simulink model "OpenLoopBallandBeam"  (R2019a)
settings: Solver=VariableStepAuto  StartTime=0.0  StopTime=10.0  RelTol=1e-3
values from neighbouring files (symbols this model uses):
  A = [0   1   0   0 ... (first row only)    [BallandBeamModeling.m]
  B = [0;  b1; 0;  0]    [BallandBeamModeling.m]
undefined symbols (not defined in the file or in its folder): K_servo
settings Model: Creator=xde12  LastModifiedBy=xde12

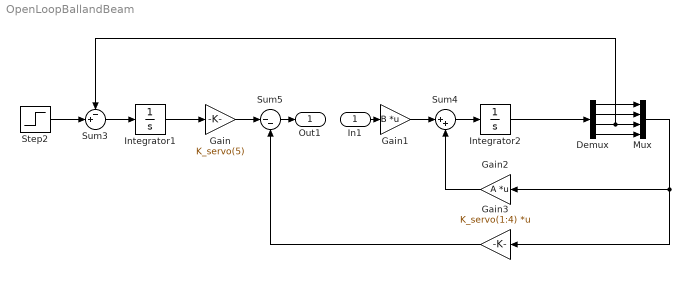
== system OpenLoopBallandBeam ==
  In1 : Inport
  Demux : Demux
  Gain : Gain  Gain=K_servo(5)
  Gain1 : Gain  Gain=B  Multiplication=Matrix(K*u)
  Gain2 : Gain  Gain=A  Multiplication=Matrix(K*u)
  Gain3 : Gain  Gain=K_servo(1:4)  Multiplication=Matrix(K*u)
  Integrator1 : Integrator
  Integrator2 : Integrator
  Mux : Mux
  Step2 : Step  Time=0  After=5  SampleTime=0.005
  Sum3 : Sum  Inputs=-+|
  Sum4 : Sum  Inputs=|++
  Sum5 : Sum  Inputs=|--
  Out1 : Outport
  wires:
  Step2/1 -> Sum3/2
  Sum3/1 -> Integrator1/1
  Integrator1/1 -> Gain/1
  Gain1/1 -> Sum4/1
  Sum4/1 -> Integrator2/1
  Gain/1 -> Sum5/1
  Gain2/1 -> Sum4/2
  Integrator2/1 -> Demux/1
  Demux/1 -> Mux/1
  Demux/2 -> Mux/2
  Demux/3 -> Sum3/1, Mux/3
  Demux/4 -> Mux/4
  Mux/1 -> Gain3/1, Gain2/1
  Gain3/1 -> Sum5/2
  Sum5/1 -> Out1/1
  In1/1 -> Gain1/1
